simulink library "csu_cmx_convert_measured_pressure_xducer_collection_lib"  (R2014b)
settings: Solver=ode45  StartTime=0.0  StopTime=10.0  RelTol=1e-3
libraries: util_info_lib x1
settings Model: Creator=escrane  LastModifiedBy=mstewart

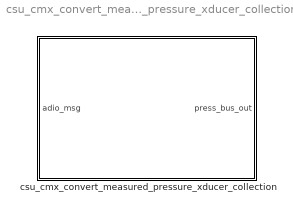
== system csu_cmx_convert_measured_pressure_xducer_collection_lib ==
  csu_cmx_convert_measured_pressure_xducer_collection : Subsystem
      mask Display: color('blue');text(0.05, 0.02, 'MoonEx', 'HorizontalAlignment', 'Left', 'VerticalAlignment', 'Bottom');color('red');text(0.95, 0.02, 'Autogenerated', 'HorizontalAlignment', 'Right', 'VerticalAlignment', 'Bottom');

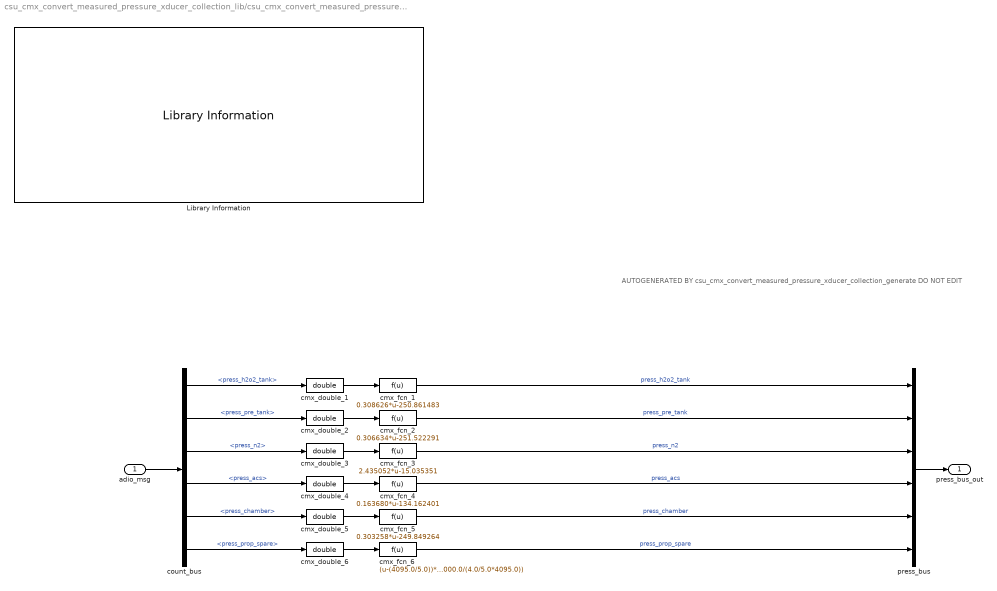
== system csu_cmx_convert_measured_pressure_xducer_collection_lib/csu_cmx_convert_measured_pressure_xducer_collection ==
  note: AUTOGENERATED BY csu_cmx_convert_measured_pressure_xducer_collection_generate
      | DO NOT EDIT
  adio_msg : Inport
  Library Information : util_info_lib/Library Information  owner='escrane'
  cmx_double_{1..6} (6 alike) : DataTypeConversion  OutDataTypeStr=double
  cmx_fcn_1 : Fcn  Expr=0.308626*u-250.861483
  cmx_fcn_2 : Fcn  Expr=0.306634*u-251.522291
  cmx_fcn_3 : Fcn  Expr=2.435052*u-15.035351
  cmx_fcn_4 : Fcn  Expr=0.163680*u-134.162401
  cmx_fcn_5 : Fcn  Expr=0.303258*u-249.849264
  cmx_fcn_6 : Fcn  Expr=(u-(4095.0/5.0))*(1000.0/(4.0/5.0*4095.0))
  count_bus : BusSelector  OutputSignals=press_h2o2_tank,press_pre_tank,press_n2,press_acs,press_chamber,press_prop_spare
  press_bus : BusCreator  Inputs=6
  press_bus_out : Outport
  wires:
  adio_msg/1 -> count_bus/1
  press_bus/1 -> press_bus_out/1
  count_bus/1 -> cmx_double_1/1  "<press_h2o2_tank>"
  cmx_double_1/1 -> cmx_fcn_1/1
  count_bus/2 -> cmx_double_2/1  "<press_pre_tank>"
  cmx_double_2/1 -> cmx_fcn_2/1
  count_bus/3 -> cmx_double_3/1  "<press_n2>"
  cmx_double_3/1 -> cmx_fcn_3/1
  cmx_fcn_3/1 -> press_bus/3  "press_n2"
  count_bus/4 -> cmx_double_4/1  "<press_acs>"
  cmx_double_4/1 -> cmx_fcn_4/1
  count_bus/5 -> cmx_double_5/1  "<press_chamber>"
  cmx_double_5/1 -> cmx_fcn_5/1
  count_bus/6 -> cmx_double_6/1  "<press_prop_spare>"
  cmx_double_6/1 -> cmx_fcn_6/1
  cmx_fcn_6/1 -> press_bus/6  "press_prop_spare"
  cmx_fcn_4/1 -> press_bus/4  "press_acs"
  cmx_fcn_5/1 -> press_bus/5  "press_chamber"
  cmx_fcn_2/1 -> press_bus/2  "press_pre_tank"
  cmx_fcn_1/1 -> press_bus/1  "press_h2o2_tank"
